simulink model "BCM2_4"  (R2021b)
settings: Solver=FixedStepDiscrete  StartTime=0.0  StopTime=1  FixedStep=0.001  RelTol=1e-3  EnableMultiTasking=on
InitFcn:
  | mbd_mpc_consistency_checks(bdroot(gcs));
model workspace (MAT data in the model file):
  CAN_rec : Simulink.Signal (value not decoded)
  CAN_transm_stat : Simulink.Signal (value not decoded)
  CAN_trm : Simulink.Signal (value not decoded)
  DITHER_CFB0 : Simulink.Parameter (value not decoded)
  DITHER_CFB1 : Simulink.Parameter (value not decoded)
  DITHER_CFB2 : Simulink.Parameter (value not decoded)
  DITHER_EN0 : Simulink.Parameter (value not decoded)
  DITHER_EN1 : Simulink.Parameter (value not decoded)
  DITHER_EN2 : Simulink.Parameter (value not decoded)
  DITHER_SIZE0 : Simulink.Parameter (value not decoded)
  DITHER_SIZE1 : Simulink.Parameter (value not decoded)
  DITHER_SIZE2 : Simulink.Parameter (value not decoded)
  DITHER_STEP0 : Simulink.Parameter (value not decoded)
  DITHER_STEP1 : Simulink.Parameter (value not decoded)
  DITHER_STEP2 : Simulink.Parameter (value not decoded)
  DITHER_SYNC0 : Simulink.Parameter (value not decoded)
  DITHER_SYNC1 : Simulink.Parameter (value not decoded)
  DITHER_SYNC2 : Simulink.Parameter (value not decoded)
  ECUMbut : Simulink.Signal (value not decoded)
  FAULTN : Simulink.Signal (value not decoded)
  FM0 : Simulink.Parameter (value not decoded)
  FM1 : Simulink.Parameter (value not decoded)
  FM2 : Simulink.Parameter (value not decoded)
  FME : Simulink.Parameter (value not decoded)
  Fsys_M : Simulink.Parameter (value not decoded)
  Fsys_N : Simulink.Parameter (value not decoded)
  Fsys_WDEN : Simulink.Parameter (value not decoded)
  Fsys_div : Simulink.Parameter (value not decoded)
  HL0 : Simulink.Parameter (value not decoded)
  HL1 : Simulink.Parameter (value not decoded)
  HL2 : Simulink.Parameter (value not decoded)
  IDIAG0 : Simulink.Parameter (value not decoded)
  IDIAG1 : Simulink.Parameter (value not decoded)
  IDIAG2 : Simulink.Parameter (value not decoded)
  Ivalve : Simulink.Signal (value not decoded)
  KI_index0 : Simulink.Parameter (value not decoded)
  KI_index1 : Simulink.Parameter (value not decoded)
  KI_index2 : Simulink.Parameter (value not decoded)
  PWM_Period0 : Simulink.Parameter (value not decoded)
  PWM_Period1 : Simulink.Parameter (value not decoded)
  PWM_Period2 : Simulink.Parameter (value not decoded)
  RESN : Simulink.Signal (value not decoded)
  SR0 : Simulink.Parameter (value not decoded)
  SR1 : Simulink.Parameter (value not decoded)
  SR2 : Simulink.Parameter (value not decoded)
  Vparam : Simulink.Signal (value not decoded)
  block_tle : Simulink.Signal (value not decoded)
  disp : Simulink.Signal (value not decoded)
  ee_adr : Simulink.Signal (value not decoded)
  ee_en_rd : Simulink.Signal (value not decoded)
  ee_en_wr : Simulink.Signal (value not decoded)
  ee_idle : Simulink.Signal (value not decoded)
  ee_read : Simulink.Signal (value not decoded)
  ee_recv : Simulink.Signal (value not decoded)
  ee_send : Simulink.Signal (value not decoded)
  in_stats : Simulink.Signal (value not decoded)
  inputs : Simulink.Signal (value not decoded)
  light : Simulink.Signal (value not decoded)
  out_drv : Simulink.Signal (value not decoded)
  out_drv_test : Simulink.Signal (value not decoded)
  out_test_en : Simulink.Signal (value not decoded)
  recv_spi2 : Simulink.Signal (value not decoded)
  ret : Simulink.Signal (value not decoded)
  spi_rcv_tle82453 : Simulink.Signal (value not decoded)
  tle82453_Ivlv : Simulink.Signal (value not decoded)
  tle82453_err : Simulink.Signal (value not decoded)
  tle82453_reset : Simulink.Signal (value not decoded)
  wtdg_CAN : Simulink.Signal (value not decoded)
symbols that are objects in the model workspace (value not decoded): CAN_rec, CAN_transm_stat, ECUMbut, inputs, Ivalve, out_drv_test, recv_spi2, ret, SR0, tle82453_Ivlv
undefined symbols (not defined in the file or in its folder): color, LQFP
libraries: simulink x68, mbd_mpc574x_ec_toolbox x50, canmsglib x42, hdlsllib x9, commutil2 x7, etargetslib x4
(part 2 of 6)

== system BCM2_4/Степы ретардера ==
  Data Store Write : DataStoreWrite  Commented=on  DataStoreName=ret  DataStoreElements=ret.step  IndexOptions=Index vector (dialog)  Indices=1  OutputSizes=1
  From2 : From  Commented=on  GotoTag=ret_stepM  TagVisibility=global
  From3 : From  Commented=on  GotoTag=ret_stepP  TagVisibility=global
  OR : Logic  Operator=OR  AllPortsSameDT=off  OutDataTypeStr=boolean
  eeprom степы ретардера : Stateflow chart  TreatAsAtomicUnit=on
      settings: PortSchema="{\"entries\":[{\"content\":{\"sides\":[{\"content\":{\"connectorIds\":[\"In1\",\"In3\",\"In2\"]},\"type\":\"ConnectorPlacement.EquallySpacedRectSide\",\"uuid\":\"1ebf9d07-d9d5-4765-a14b-d01132fae39d\"},{\"content\":{\"connectorIds\":[],\"side\":\"RIGHT\"},\"type\":\"ConnectorPlacement.EquallySpacedRectSide\",\"uuid\":\"961b2fe5-8f90-4192-8201-219491ef069e\"},{\"content\":{\"connectorIds\":[],\"side\":\"TOP\"},\"type\":\"ConnectorPlacement.EquallySpacedRectSide\",\"uuid\":\"9050879b-edec-4af7-9289-aadedb2c5dee\"}]},\"type\":\"ConnectorPlacement.EquallySpacedConnector\",\"uuid\":\"75c99b9c-2e9d-4193-9189-f6fceb65a5f8\"}],\"packageUris\":[\"http://schema.mathworks.com/mf0/Connector/R2020b\"],\"version\":\"1.0\"}"
  Степы ретардера : Stateflow chart  Commented=on  TreatAsAtomicUnit=on
  страницы механика+ : Subsystem  TreatAsAtomicUnit=on
  страницы механика- : Subsystem  TreatAsAtomicUnit=on
  wires:
  From2/1 -> Степы ретардера/1(stepM)
  Степы ретардера/1(Step_ret) -> Data Store Write/1
  From3/1 -> Степы ретардера/2(stepP)
  [ret_stepM] -> OR/1, страницы механика-/Trigger
  OR/1 -> eeprom степы ретардера/1(write_ee)
  [ret_stepP] -> страницы механика+/Trigger, OR/2
  страницы механика+/1(Out_max_ret) -> eeprom степы ретардера/3(step_max)
  страницы механика+/2(Out_max_brk) -> eeprom степы ретардера/2(step_brk_max)

== system BCM2_4/Топливные баки ==
  Pump1 : Inport
  Pump2 : Inport  Port=2
  rashod : Inport  Port=3
  Compare To Constant : simulink/Logic and Bit Operations/Compare To Constant  relop=>  const=0  OutDataTypeStr=boolean
  Data Store Memory : DataStoreMemory  DataStoreName=tank1  ReadBeforeWriteMsg=warning  WriteAfterWriteMsg=warning  WriteAfterReadMsg=warning  InitialValue=ft1  ShowAdditionalParam=off
  Data Store Memory1 : DataStoreMemory  DataStoreName=tank2  ReadBeforeWriteMsg=warning  WriteAfterWriteMsg=warning  WriteAfterReadMsg=warning  InitialValue=ft2  ShowAdditionalParam=off
  Data Store Memory2 : DataStoreMemory  DataStoreName=tank3  ReadBeforeWriteMsg=warning  WriteAfterWriteMsg=warning  WriteAfterReadMsg=warning  InitialValue=ft3  ShowAdditionalParam=off
  Data Store Read : DataStoreRead  DataStoreName=tank3  IndexOptions=Index vector (dialog)  Indices=1  OutputSizes=1
  Data Store Read4 : DataStoreRead  DataStoreName=tank1  IndexOptions=Index vector (dialog)  Indices=1  OutputSizes=1
  Data Store Read5 : DataStoreRead  DataStoreName=tank2  IndexOptions=Index vector (dialog)  Indices=1  OutputSizes=1
  Data Store Read6 : DataStoreRead  DataStoreName=tank3  IndexOptions=Index vector (dialog)  Indices=1  OutputSizes=1
  Enabled Subsystem : Subsystem  TreatAsAtomicUnit=on
  Enabled Subsystem1 : Subsystem  TreatAsAtomicUnit=on
  Subsystem : Subsystem
  Tank1 : Outport
  Tank2 : Outport  Port=2
  Tank3 : Outport  Port=3
  wires:
  Pump1/1 -> Enabled Subsystem/Enable
  Pump2/1 -> Enabled Subsystem1/Enable
  Data Store Read4/1 -> Tank1/1
  Data Store Read5/1 -> Tank2/1
  Data Store Read6/1 -> Tank3/1
  rashod/1 -> Subsystem/1(In1)
  Data Store Read/1 -> Compare To Constant/1
  Compare To Constant/1 -> Subsystem/Enable

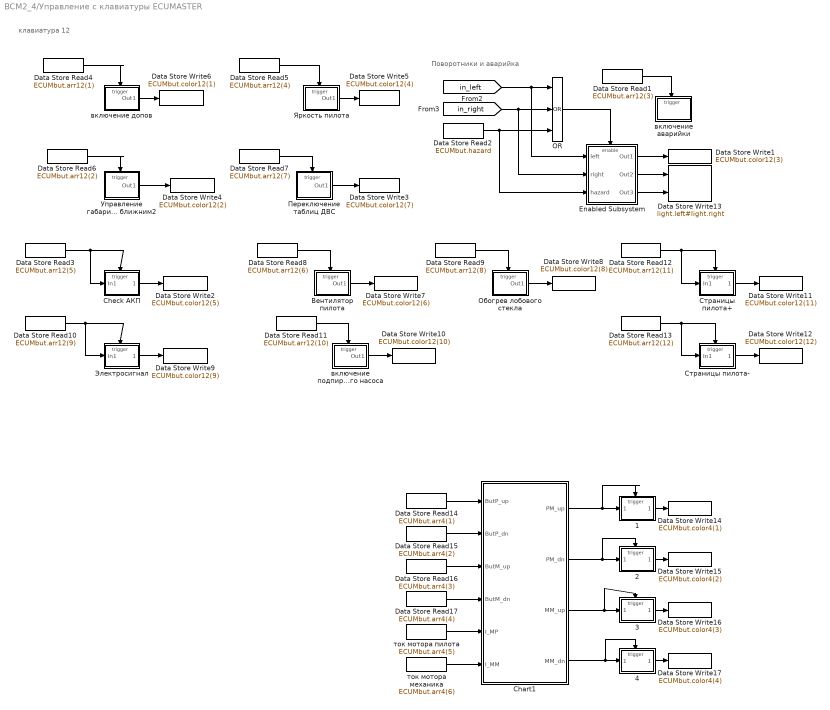
== system BCM2_4/Управление с клавиатуры ECUMASTER ==
  note: клавиатура 12
  note: Поворотники и аварийка
  1 : Subsystem
  2 : Subsystem
  3 : Subsystem
  4 : Subsystem
  Chart1 : Stateflow chart  TreatAsAtomicUnit=on
  Check АКП : Subsystem
  Data Store Read1 : DataStoreRead  DataStoreName=ECUMbut  DataStoreElements=ECUMbut.arr12(3)  IndexOptions=Index vector (dialog)  Indices=1  OutputSizes=1
  Data Store Read10 : DataStoreRead  DataStoreName=ECUMbut  DataStoreElements=ECUMbut.arr12(9)  IndexOptions=Index vector (dialog)  Indices=1  OutputSizes=1
  Data Store Read11 : DataStoreRead  DataStoreName=ECUMbut  DataStoreElements=ECUMbut.arr12(10)  IndexOptions=Index vector (dialog)  Indices=1  OutputSizes=1
  Data Store Read12 : DataStoreRead  DataStoreName=ECUMbut  DataStoreElements=ECUMbut.arr12(11)  IndexOptions=Index vector (dialog)  Indices=1  OutputSizes=1
  Data Store Read13 : DataStoreRead  DataStoreName=ECUMbut  DataStoreElements=ECUMbut.arr12(12)  IndexOptions=Index vector (dialog)  Indices=1  OutputSizes=1
  Data Store Read14 : DataStoreRead  DataStoreName=ECUMbut  DataStoreElements=ECUMbut.arr4(1)  IndexOptions=Index vector (dialog)  Indices=1  OutputSizes=1
  Data Store Read15 : DataStoreRead  DataStoreName=ECUMbut  DataStoreElements=ECUMbut.arr4(2)  IndexOptions=Index vector (dialog)  Indices=1  OutputSizes=1
  Data Store Read16 : DataStoreRead  DataStoreName=ECUMbut  DataStoreElements=ECUMbut.arr4(3)  IndexOptions=Index vector (dialog)  Indices=1  OutputSizes=1
  Data Store Read17 : DataStoreRead  DataStoreName=ECUMbut  DataStoreElements=ECUMbut.arr4(4)  IndexOptions=Index vector (dialog)  Indices=1  OutputSizes=1
  Data Store Read2 : DataStoreRead  DataStoreName=ECUMbut  DataStoreElements=ECUMbut.hazard  IndexOptions=Index vector (dialog)  Indices=1  OutputSizes=1
  Data Store Read3 : DataStoreRead  DataStoreName=ECUMbut  DataStoreElements=ECUMbut.arr12(5)  IndexOptions=Index vector (dialog)  Indices=1  OutputSizes=1
  Data Store Read4 : DataStoreRead  DataStoreName=ECUMbut  DataStoreElements=ECUMbut.arr12(1)  IndexOptions=Index vector (dialog)  Indices=1  OutputSizes=1
  Data Store Read5 : DataStoreRead  DataStoreName=ECUMbut  DataStoreElements=ECUMbut.arr12(4)  IndexOptions=Index vector (dialog)  Indices=1  OutputSizes=1
  Data Store Read6 : DataStoreRead  DataStoreName=ECUMbut  DataStoreElements=ECUMbut.arr12(2)  IndexOptions=Index vector (dialog)  Indices=1  OutputSizes=1
  Data Store Read7 : DataStoreRead  DataStoreName=ECUMbut  DataStoreElements=ECUMbut.arr12(7)  IndexOptions=Index vector (dialog)  Indices=1  OutputSizes=1
  Data Store Read8 : DataStoreRead  DataStoreName=ECUMbut  DataStoreElements=ECUMbut.arr12(6)  IndexOptions=Index vector (dialog)  Indices=1  OutputSizes=1
  Data Store Read9 : DataStoreRead  DataStoreName=ECUMbut  DataStoreElements=ECUMbut.arr12(8)  IndexOptions=Index vector (dialog)  Indices=1  OutputSizes=1
  Data Store Write1 : DataStoreWrite  DataStoreName=ECUMbut  DataStoreElements=ECUMbut.color12(3)  IndexOptions=Index vector (dialog)  Indices=1  OutputSizes=1
  Data Store Write10 : DataStoreWrite  DataStoreName=ECUMbut  DataStoreElements=ECUMbut.color12(10)  IndexOptions=Index vector (dialog)  Indices=1  OutputSizes=1
  Data Store Write11 : DataStoreWrite  DataStoreName=ECUMbut  DataStoreElements=ECUMbut.color12(11)  IndexOptions=Index vector (dialog)  Indices=1  OutputSizes=1
  Data Store Write12 : DataStoreWrite  DataStoreName=ECUMbut  DataStoreElements=ECUMbut.color12(12)  IndexOptions=Index vector (dialog)  Indices=1  OutputSizes=1
  Data Store Write13 : DataStoreWrite  DataStoreName=light  DataStoreElements=light.left#light.right  IndexOptions=Index vector (dialog)  Indices=1  OutputSizes=1
  Data Store Write14 : DataStoreWrite  DataStoreName=ECUMbut  DataStoreElements=ECUMbut.color4(1)  IndexOptions=Index vector (dialog)  Indices=1  OutputSizes=1
  Data Store Write15 : DataStoreWrite  DataStoreName=ECUMbut  DataStoreElements=ECUMbut.color4(2)  IndexOptions=Index vector (dialog)  Indices=1  OutputSizes=1
  Data Store Write16 : DataStoreWrite  DataStoreName=ECUMbut  DataStoreElements=ECUMbut.color4(3)  IndexOptions=Index vector (dialog)  Indices=1  OutputSizes=1
  Data Store Write17 : DataStoreWrite  DataStoreName=ECUMbut  DataStoreElements=ECUMbut.color4(4)  IndexOptions=Index vector (dialog)  Indices=1  OutputSizes=1
  Data Store Write2 : DataStoreWrite  DataStoreName=ECUMbut  DataStoreElements=ECUMbut.color12(5)  IndexOptions=Index vector (dialog)  Indices=1  OutputSizes=1
  Data Store Write3 : DataStoreWrite  DataStoreName=ECUMbut  DataStoreElements=ECUMbut.color12(7)  IndexOptions=Index vector (dialog)  Indices=1  OutputSizes=1
  Data Store Write4 : DataStoreWrite  DataStoreName=ECUMbut  DataStoreElements=ECUMbut.color12(2)  IndexOptions=Index vector (dialog)  Indices=1  OutputSizes=1
  Data Store Write5 : DataStoreWrite  DataStoreName=ECUMbut  DataStoreElements=ECUMbut.color12(4)  IndexOptions=Index vector (dialog)  Indices=1  OutputSizes=1
  Data Store Write6 : DataStoreWrite  DataStoreName=ECUMbut  DataStoreElements=ECUMbut.color12(1)  IndexOptions=Index vector (dialog)  Indices=1  OutputSizes=1
  Data Store Write7 : DataStoreWrite  DataStoreName=ECUMbut  DataStoreElements=ECUMbut.color12(6)  IndexOptions=Index vector (dialog)  Indices=1  OutputSizes=1
  Data Store Write8 : DataStoreWrite  DataStoreName=ECUMbut  DataStoreElements=ECUMbut.color12(8)  IndexOptions=Index vector (dialog)  Indices=1  OutputSizes=1
  Data Store Write9 : DataStoreWrite  DataStoreName=ECUMbut  DataStoreElements=ECUMbut.color12(9)  IndexOptions=Index vector (dialog)  Indices=1  OutputSizes=1
  Enabled Subsystem : Subsystem  TreatAsAtomicUnit=on
  OR : Logic  Operator=OR  Inputs=3  AllPortsSameDT=off  OutDataTypeStr=boolean
  Вентилятор пилота : Subsystem
  Обогрев лобового стекла : Subsystem
  Переключение таблиц ДВС : Subsystem  TreatAsAtomicUnit=on
  Страницы пилота+ : Subsystem
  Страницы пилота- : Subsystem
  Управление габаритами и ближним2 : Subsystem  TreatAsAtomicUnit=on
  Электросигнал : Subsystem
  Яркость пилота : Subsystem
  включение аварийки : Subsystem
  включение допов : Subsystem
  включение подпирающего топливного насоса : Subsystem
  ток мотора механика : DataStoreRead  DataStoreName=ECUMbut  DataStoreElements=ECUMbut.arr4(6)  IndexOptions=Index vector (dialog)  Indices=1  OutputSizes=1
  ток мотора пилота : DataStoreRead  DataStoreName=ECUMbut  DataStoreElements=ECUMbut.arr4(5)  IndexOptions=Index vector (dialog)  Indices=1  OutputSizes=1
  wires:
  Data Store Read4/1 -> включение допов/Trigger
  Яркость пилота/1(Out1) -> Data Store Write5/1
  Data Store Read7/1 -> Переключение таблиц ДВС/Trigger
  Data Store Read5/1 -> Яркость пилота/Trigger
  Управление габаритами и ближним2/1(Out1) -> Data Store Write4/1
  включение допов/1(Out1) -> Data Store Write6/1
  Переключение таблиц ДВС/1(Out1) -> Data Store Write3/1
  Data Store Read6/1 -> Управление габаритами и ближним2/Trigger
  Data Store Read1/1 -> включение аварийки/Trigger
  [in_left] -> Enabled Subsystem/1(left), OR/1
  [in_right] -> Enabled Subsystem/2(right), OR/2
  Data Store Read2/1 -> Enabled Subsystem/3(hazard), OR/3
  OR/1 -> Enabled Subsystem/Enable
  Enabled Subsystem/1(Out1) -> Data Store Write1/1
  Check АКП/1(Out1) -> Data Store Write2/1
  Data Store Read3/1 -> Check АКП/1(In1), Check АКП/Trigger
  Вентилятор пилота/1(Out1) -> Data Store Write7/1
  Data Store Read8/1 -> Вентилятор пилота/Trigger
  Обогрев лобового стекла/1(Out1) -> Data Store Write8/1
  Data Store Read9/1 -> Обогрев лобового стекла/Trigger
  Data Store Read10/1 -> Электросигнал/1(In1), Электросигнал/Trigger
  Электросигнал/1(Out1) -> Data Store Write9/1
  включение подпирающего топливного насоса/1(Out1) -> Data Store Write10/1
  Data Store Read11/1 -> включение подпирающего топливного насоса/Trigger
  Страницы пилота+/1(Out1) -> Data Store Write11/1
  Data Store Read12/1 -> Страницы пилота+/Trigger, Страницы пилота+/1(In1)
  Data Store Read13/1 -> Страницы пилота-/1(In1), Страницы пилота-/Trigger
  Страницы пилота-/1(Out1) -> Data Store Write12/1
  Enabled Subsystem/2(Out2) -> Data Store Write13/1
  Enabled Subsystem/3(Out3) -> Data Store Write13/2
  1/1(Out1) -> Data Store Write14/1
  ток мотора пилота/1 -> Chart1/5(I_MP)
  ток мотора механика/1 -> Chart1/6(I_MM)
  Chart1/1(PM_up) -> 1/1(PM_up), 1/Trigger
  2/1(Out1) -> Data Store Write15/1
  3/1(Out1) -> Data Store Write16/1
  4/1(Out1) -> Data Store Write17/1
  Chart1/2(PM_dn) -> 2/Trigger, 2/1(PM_up)
  Chart1/3(MM_up) -> 3/1(PM_up), 3/Trigger
  Chart1/4(MM_dn) -> 4/1(PM_up), 4/Trigger
  Data Store Read14/1 -> Chart1/1(ButP_up)
  Data Store Read15/1 -> Chart1/2(ButP_dn)
  Data Store Read16/1 -> Chart1/3(ButM_up)
  Data Store Read17/1 -> Chart1/4(ButM_dn)

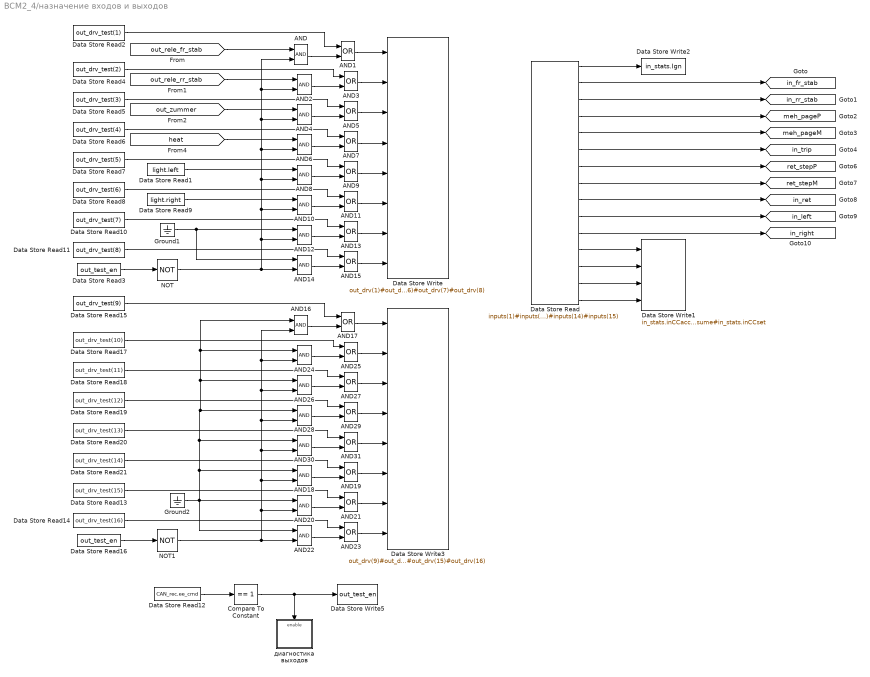
== system BCM2_4/назначение входов и выходов ==
  AND{,2,4,6,8,10,12,14,16,18,20,22,24,26,28,30} (16 alike) : Logic  AllPortsSameDT=off  OutDataTypeStr=boolean
  AND{1,3,5,7,9,11,13,15,17,19,21,23,25,27,29,31} (16 alike) : Logic  Operator=OR  AllPortsSameDT=off  OutDataTypeStr=boolean
  Compare To Constant : simulink/Logic and Bit Operations/Compare To Constant  relop===  const=1  OutDataTypeStr=boolean
  Data Store Read : DataStoreRead  DataStoreName=inputs  DataStoreElements=inputs(1)#inputs(2)#inputs(3)#inputs(4)#inputs(5)#inputs(6)#inputs(7)#inputs(8)#inputs(9)#inputs(10)#inputs(11)#inputs(12)#inputs(13)#inputs(14)#inputs(15)  IndexOptions=Index vector (dialog)  Indices=1  OutputSizes=1
  Data Store Read1 : DataStoreRead  DataStoreName=light  DataStoreElements=light.left  IndexOptions=Index vector (dialog)  Indices=1  OutputSizes=1
  Data Store Read10 : DataStoreRead  DataStoreName=out_drv_test  DataStoreElements=out_drv_test(7)  IndexOptions=Index vector (dialog)  Indices=1  OutputSizes=1
  Data Store Read11 : DataStoreRead  DataStoreName=out_drv_test  DataStoreElements=out_drv_test(8)  IndexOptions=Index vector (dialog)  Indices=1  OutputSizes=1
  Data Store Read12 : DataStoreRead  DataStoreName=CAN_rec  SampleTime=0.1  DataStoreElements=CAN_rec.ee_cmd  IndexOptions=Index vector (dialog)  Indices=1  OutputSizes=1
  Data Store Read13 : DataStoreRead  DataStoreName=out_drv_test  DataStoreElements=out_drv_test(15)  IndexOptions=Index vector (dialog)  Indices=1  OutputSizes=1
  Data Store Read14 : DataStoreRead  DataStoreName=out_drv_test  DataStoreElements=out_drv_test(16)  IndexOptions=Index vector (dialog)  Indices=1  OutputSizes=1
  Data Store Read15 : DataStoreRead  DataStoreName=out_drv_test  DataStoreElements=out_drv_test(9)  IndexOptions=Index vector (dialog)  Indices=1  OutputSizes=1
  Data Store Read16 : DataStoreRead  DataStoreName=out_test_en  IndexOptions=Index vector (dialog)  Indices=1  OutputSizes=1
  Data Store Read17 : DataStoreRead  DataStoreName=out_drv_test  DataStoreElements=out_drv_test(10)  IndexOptions=Index vector (dialog)  Indices=1  OutputSizes=1
  Data Store Read18 : DataStoreRead  DataStoreName=out_drv_test  DataStoreElements=out_drv_test(11)  IndexOptions=Index vector (dialog)  Indices=1  OutputSizes=1
  Data Store Read19 : DataStoreRead  DataStoreName=out_drv_test  DataStoreElements=out_drv_test(12)  IndexOptions=Index vector (dialog)  Indices=1  OutputSizes=1
  Data Store Read2 : DataStoreRead  DataStoreName=out_drv_test  DataStoreElements=out_drv_test(1)  IndexOptions=Index vector (dialog)  Indices=1  OutputSizes=1
  Data Store Read20 : DataStoreRead  DataStoreName=out_drv_test  DataStoreElements=out_drv_test(13)  IndexOptions=Index vector (dialog)  Indices=1  OutputSizes=1
  Data Store Read21 : DataStoreRead  DataStoreName=out_drv_test  DataStoreElements=out_drv_test(14)  IndexOptions=Index vector (dialog)  Indices=1  OutputSizes=1
  Data Store Read3 : DataStoreRead  DataStoreName=out_test_en  IndexOptions=Index vector (dialog)  Indices=1  OutputSizes=1
  Data Store Read4 : DataStoreRead  DataStoreName=out_drv_test  DataStoreElements=out_drv_test(2)  IndexOptions=Index vector (dialog)  Indices=1  OutputSizes=1
  Data Store Read5 : DataStoreRead  DataStoreName=out_drv_test  DataStoreElements=out_drv_test(3)  IndexOptions=Index vector (dialog)  Indices=1  OutputSizes=1
  Data Store Read6 : DataStoreRead  DataStoreName=out_drv_test  DataStoreElements=out_drv_test(4)  IndexOptions=Index vector (dialog)  Indices=1  OutputSizes=1
  Data Store Read7 : DataStoreRead  DataStoreName=out_drv_test  DataStoreElements=out_drv_test(5)  IndexOptions=Index vector (dialog)  Indices=1  OutputSizes=1
  Data Store Read8 : DataStoreRead  DataStoreName=out_drv_test  DataStoreElements=out_drv_test(6)  IndexOptions=Index vector (dialog)  Indices=1  OutputSizes=1
  Data Store Read9 : DataStoreRead  DataStoreName=light  DataStoreElements=light.right  IndexOptions=Index vector (dialog)  Indices=1  OutputSizes=1
  Data Store Write : DataStoreWrite  DataStoreName=out_drv  DataStoreElements=out_drv(1)#out_drv(2)#out_drv(3)#out_drv(4)#out_drv(5)#out_drv(6)#out_drv(7)#out_drv(8)  IndexOptions=Index vector (dialog)  Indices=1  OutputSizes=1
  Data Store Write1 : DataStoreWrite  DataStoreName=in_stats  DataStoreElements=in_stats.inCCacc#in_stats.inCCcoast#in_stats.inCCresume#in_stats.inCCset  IndexOptions=Index vector (dialog)  Indices=1  OutputSizes=1
  Data Store Write2 : DataStoreWrite  DataStoreName=in_stats  DataStoreElements=in_stats.Ign  IndexOptions=Index vector (dialog)  Indices=1  OutputSizes=1
  Data Store Write3 : DataStoreWrite  DataStoreName=out_drv  SampleTime=0.01  DataStoreElements=out_drv(9)#out_drv(10)#out_drv(11)#out_drv(12)#out_drv(13)#out_drv(14)#out_drv(15)#out_drv(16)  IndexOptions=Index vector (dialog)  Indices=1  OutputSizes=1
  Data Store Write5 : DataStoreWrite  DataStoreName=out_test_en  IndexOptions=Index vector (dialog)  Indices=1  OutputSizes=1
  Ground1 : Ground
  Ground2 : Ground
  NOT : Logic  Operator=NOT  IconShape=distinctive  AllPortsSameDT=off  OutDataTypeStr=boolean
  NOT1 : Logic  Operator=NOT  IconShape=distinctive  AllPortsSameDT=off  OutDataTypeStr=boolean
  диагностика выходов : Subsystem
  tag scope: in_fr_stab=global, in_left=global, in_ret=global, in_right=global, in_rr_stab=global, in_trip=global, meh_pageM=global, meh_pageP=global, ret_stepM=global, ret_stepP=global
  wires:
  Data Store Read/5 -> [meh_pageM]
  Data Store Read/6 -> [in_trip]
  Data Store Read/7 -> [ret_stepP]
  Data Store Read/8 -> [ret_stepM]
  Data Store Read/9 -> [in_ret]
  Data Store Read/10 -> [in_left]
  Data Store Read/11 -> [in_right]
  [out_rele_fr_stab] -> AND/1
  [out_rele_rr_stab] -> AND2/1
  [out_zummer] -> AND4/1
  Ground1/1 -> AND12/1, AND14/1
  [heat] -> AND6/1
  Data Store Read1/1 -> AND8/1
  Data Store Read9/1 -> AND10/1
  Data Store Read/12 -> Data Store Write1/1
  Data Store Read/13 -> Data Store Write1/2
  Data Store Read/14 -> Data Store Write1/3
  Data Store Read/15 -> Data Store Write1/4
  Data Store Read/1 -> Data Store Write2/1
  Data Store Read/2 -> [in_fr_stab]
  Data Store Read/3 -> [in_rr_stab]
  Data Store Read/4 -> [meh_pageP]
  AND1/1 -> Data Store Write/1
  AND/1 -> AND1/2
  AND2/1 -> AND3/2
  AND3/1 -> Data Store Write/2
  AND4/1 -> AND5/2
  AND5/1 -> Data Store Write/3
  AND6/1 -> AND7/2
  AND7/1 -> Data Store Write/4
  AND8/1 -> AND9/2
  AND9/1 -> Data Store Write/5
  AND10/1 -> AND11/2
  AND11/1 -> Data Store Write/6
  AND12/1 -> AND13/2
  AND13/1 -> Data Store Write/7
  AND14/1 -> AND15/2
  AND15/1 -> Data Store Write/8
  Data Store Read3/1 -> NOT/1
  Data Store Read2/1 -> AND1/1
  Data Store Read4/1 -> AND3/1
  Data Store Read5/1 -> AND5/1
  Data Store Read6/1 -> AND7/1
  Data Store Read7/1 -> AND9/1
  Data Store Read8/1 -> AND11/1
  Data Store Read10/1 -> AND13/1
  Data Store Read11/1 -> AND15/1
  Data Store Read14/1 -> AND23/1
  Data Store Read13/1 -> AND21/1
  Data Store Read21/1 -> AND19/1
  Data Store Read20/1 -> AND31/1
  Data Store Read19/1 -> AND29/1
  Data Store Read18/1 -> AND27/1
  Data Store Read17/1 -> AND25/1
  Data Store Read15/1 -> AND17/1
  Data Store Read16/1 -> NOT1/1
  AND23/1 -> Data Store Write3/8
  AND22/1 -> AND23/2
  AND21/1 -> Data Store Write3/7
  AND20/1 -> AND21/2
  AND19/1 -> Data Store Write3/6
  AND18/1 -> AND19/2
  AND31/1 -> Data Store Write3/5
  AND30/1 -> AND31/2
  AND29/1 -> Data Store Write3/4
  AND28/1 -> AND29/2
  AND27/1 -> Data Store Write3/3
  AND26/1 -> AND27/2
  AND25/1 -> Data Store Write3/2
  AND24/1 -> AND25/2
  AND16/1 -> AND17/2
  AND17/1 -> Data Store Write3/1
  Ground2/1 -> AND22/1, AND16/1, AND24/1, AND26/1, AND28/1, AND30/1, AND18/1, AND20/1
  NOT/1 -> AND14/2, AND12/2, AND10/2, AND8/2, AND6/2, AND4/2, AND2/2, AND/2
  NOT1/1 -> AND16/2, AND24/2, AND26/2, AND28/2, AND30/2, AND18/2, AND20/2, AND22/2
  Compare To Constant/1 -> Data Store Write5/1, диагностика выходов/Enable
  Data Store Read12/1 -> Compare To Constant/1

== system BCM2_4/управление лепестками ==
  Data Store Write : DataStoreWrite  DataStoreName=ret  DataStoreElements=ret.ret_en  IndexOptions=Index vector (dialog)  Indices=1  OutputSizes=1
  Remote stab : Stateflow chart  TreatAsAtomicUnit=on
  tag scope: out_rele_fr_stab=global, out_rele_rr_stab=global, out_zummer=global
  wires:
  [in_fr_stab] -> Remote stab/1(sw_fr_stab)
  Remote stab/3(zummer) -> [out_zummer]
  Remote stab/2(rele_rr_stab) -> [out_rele_rr_stab]
  Remote stab/1(rele_fr_stab) -> [out_rele_fr_stab]
  [in_rr_stab] -> Remote stab/2(sw_rr_stab)
  Remote stab/4(rele_ret) -> Data Store Write/1
  [in_ret] -> Remote stab/3(sw_ret)

== system BCM2_4/управление страницами и яркостью мониторов ==
  Constant : Constant  OutDataTypeStr=boolean
  Data Store Read1 : DataStoreRead  DataStoreName=ECUMbut  DataStoreElements=ECUMbut.bright_pilot  IndexOptions=Index vector (dialog)  Indices=1  OutputSizes=1
  Data Store Read2 : DataStoreRead  DataStoreName=CAN_trm  DataStoreElements=CAN_trm.wPilotPageP#CAN_trm.wPilotPageM  IndexOptions=Index vector (dialog)  Indices=1  OutputSizes=1
  Data Store Read4 : DataStoreRead  DataStoreName=ECUMbut  DataStoreElements=ECUMbut.PageP#ECUMbut.PageM  IndexOptions=Index vector (dialog)  Indices=1  OutputSizes=1
  Display : Display
  Display1 : Display
  OR : Logic  Operator=OR  Inputs=4  AllPortsSameDT=off  OutDataTypeStr=boolean
  OR1 : Logic  Operator=OR  AllPortsSameDT=off  OutDataTypeStr=boolean
  OR2 : Logic  Operator=OR  AllPortsSameDT=off  OutDataTypeStr=boolean
  Remote bright : Stateflow chart  TreatAsAtomicUnit=on
      settings: PortSchema="{\"entries\":[{\"content\":{\"sides\":[{\"content\":{\"connectorIds\":[\"In2\",\"In1\"]},\"type\":\"ConnectorPlacement.EquallySpacedRectSide\",\"uuid\":\"b649a9c8-237f-4f0e-8c49-622a9c826017\"},{\"content\":{\"connectorIds\":[\"Out1\",\"Out2\"],\"side\":\"RIGHT\"},\"type\":\"ConnectorPlacement.EquallySpacedRectSide\",\"uuid\":\"0d804784-30f9-473e-82b5-002cce05e2f2\"},{\"content\":{\"connectorIds\":[],\"side\":\"TOP\"},\"type\":\"ConnectorPlacement.EquallySpacedRectSide\",\"uuid\":\"6d8957c1-8347-4a30-84c4-fd66e5fe6d42\"},{\"content\":{\"connectorIds\":[],\"side\":\"HIDDEN\"},\"type\":\"ConnectorPlacement.EquallySpacedRectSide\",\"uuid\":\"9712d6bb-fd29-4f07-870a-122e6c317742\"}]},\"type\":\"ConnectorPlacement.EquallySpacedConnector\",\"uuid\":\"dcd1749c-602d-455d-8651-1ffb4d1b2b2f\"}],\"packageUris\":[\"http://schema.mathworks.com/mf0/Connector/R2020b\"],\"version\":\"1.0\"}"
  eeprom страницы : Stateflow chart  TreatAsAtomicUnit=on
  страницы механика+ : Subsystem  TreatAsAtomicUnit=on
  страницы механика- : Subsystem  TreatAsAtomicUnit=on
  страницы пилота+ : Subsystem  TreatAsAtomicUnit=on
  страницы пилота- : Subsystem  TreatAsAtomicUnit=on
  wires:
  Constant/1 -> Remote bright/1(inM)
  Remote bright/1(outP) -> Display/1
  Remote bright/2(outM) -> Display1/1
  Data Store Read1/1 -> Remote bright/2(inP)
  [meh_pageP] -> страницы механика+/Trigger, OR/3
  [meh_pageM] -> страницы механика-/Trigger, OR/4
  OR2/1 -> страницы пилота-/Trigger, OR/2
  OR/1 -> eeprom страницы/1(write_ee)
  OR1/1 -> страницы пилота+/Trigger, OR/1
  Data Store Read4/1 -> OR1/2
  Data Store Read2/1 -> OR1/1
  Data Store Read4/2 -> OR2/1
  Data Store Read2/2 -> OR2/2

== system BCM2_4/CAN WATCHDOG/wtdg CCVS1_00 ==
  function : TriggerPort  TriggerType=function-call  VariantControl=(inherit)
  Constant : Constant  Value=0
  Data Store Write4 : DataStoreWrite  DataStoreName=Vparam  DataStoreElements=Vparam.Vspd  IndexOptions=Index vector (dialog)  Indices=1  OutputSizes=1
  wires:
  Constant/1 -> Data Store Write4/1

== system BCM2_4/CAN WATCHDOG/wtdg EBC1 ==
  function : TriggerPort  TriggerType=function-call  VariantControl=(inherit)
  Constant : Constant  Value=0  OutDataTypeStr=uint8
  Data Store Write : DataStoreWrite  DataStoreName=Vparam  DataStoreElements=Vparam.BrakePos  IndexOptions=Index vector (dialog)  Indices=1  OutputSizes=1
  wires:
  Constant/1 -> Data Store Write/1

== system BCM2_4/CAN WATCHDOG/wtdg EEC1_300 ==
  function : TriggerPort  TriggerType=function-call  VariantControl=(inherit)
  Constant : Constant  Value=0  OutDataTypeStr=uint8
  Data Store Write : DataStoreWrite  DataStoreName=Vparam  DataStoreElements=Vparam.PedalPos  IndexOptions=Index vector (dialog)  Indices=1  OutputSizes=1
  wires:
  Constant/1 -> Data Store Write/1

== system BCM2_4/CAN WATCHDOG/wtdg EEC1_400 ==
  function : TriggerPort  TriggerType=function-call  VariantControl=(inherit)
  Constant : Constant  Value=0  OutDataTypeStr=uint16
  Data Store Write : DataStoreWrite  DataStoreName=Vparam  DataStoreElements=Vparam.Espd  IndexOptions=Index vector (dialog)  Indices=1  OutputSizes=1
  wires:
  Constant/1 -> Data Store Write/1

== system BCM2_4/CAN WATCHDOG/wtdg ETC1 ==
  function : TriggerPort  TriggerType=function-call  VariantControl=(inherit)

== system BCM2_4/CAN WATCHDOG/wtdg FuelTank ==
  function : TriggerPort  TriggerType=function-call  VariantControl=(inherit)

== system BCM2_4/CAN WATCHDOG/wtdg RF ==
  function : TriggerPort  TriggerType=function-call  VariantControl=(inherit)
  Constant : Constant  Value=180
  Data Store Write : DataStoreWrite  DataStoreName=ret  DataStoreElements=ret.RetTemp  IndexOptions=Index vector (dialog)  Indices=1  OutputSizes=1
  wires:
  Constant/1 -> Data Store Write/1

== system BCM2_4/CAN WATCHDOG/wtdg VD ==
  function : TriggerPort  TriggerType=function-call  VariantControl=(inherit)

== system BCM2_4/CAN WATCHDOG/wtdg ee_wr ==
  function : TriggerPort  TriggerType=function-call  VariantControl=(inherit)
  Constant1 : Constant  Value=0  OutDataTypeStr=boolean
  Constant2 : Constant  Value=0  OutDataTypeStr=uint8
  Data Store Write2 : DataStoreWrite  DataStoreName=CAN_rec  DataStoreElements=CAN_rec.ee_rec_stat  IndexOptions=Index vector (dialog)  Indices=1  OutputSizes=1
  Data Store Write4 : DataStoreWrite  DataStoreName=CAN_rec  DataStoreElements=CAN_rec.ee_cmd  IndexOptions=Index vector (dialog)  Indices=1  OutputSizes=1
  wires:
  Constant1/1 -> Data Store Write2/1
  Constant2/1 -> Data Store Write4/1

== system BCM2_4/CAN WATCHDOG/wtdg id101 ==
  function : TriggerPort  TriggerType=function-call  VariantControl=(inherit)

== system BCM2_4/CAN WATCHDOG/wtdg id192 ==
  function : TriggerPort  TriggerType=function-call  VariantControl=(inherit)

== system BCM2_4/CAN WATCHDOG/wtdg id195 ==
  function : TriggerPort  TriggerType=function-call  VariantControl=(inherit)
  Constant : Constant  Value=[0 0 0 0 0 0 0 0 0 0 0 0 0 0 0 0]  OutDataTypeStr=boolean
  Data Store Write : DataStoreWrite  DataStoreName=ECUMbut  DataStoreElements=ECUMbut.arr12(:)  IndexOptions=Index vector (dialog)  Indices=1  OutputSizes=1
  wires:
  Constant/1 -> Data Store Write/1

== system BCM2_4/CAN WATCHDOG/wtdg max_page_meh ==
  function : TriggerPort  TriggerType=function-call  VariantControl=(inherit)

== system BCM2_4/CAN WATCHDOG/wtdg max_page_pilot ==
  function : TriggerPort  TriggerType=function-call  VariantControl=(inherit)

== system BCM2_4/CAN WATCHDOG/wtdg w18F0010B ==
  function : TriggerPort  TriggerType=function-call  VariantControl=(inherit)

== system BCM2_4/CAN WATCHDOG/wtdg w18FEAD0B ==
  function : TriggerPort  TriggerType=function-call  VariantControl=(inherit)

== system BCM2_4/CAN WATCHDOG/wtdg w18FEEA2F ==
  function : TriggerPort  TriggerType=function-call  VariantControl=(inherit)

== system BCM2_4/CAN0 Transmit buf 5-21/0CFED911 AUXIO buf = 11 ==
  Enable : EnablePort
  0CFED911 AUXIO buf = 11 : Subsystem  TreatAsAtomicUnit=on  SystemSampleTime=0.1

== system BCM2_4/CAN0 Transmit buf 5-21/0CFEF111 CCVS1 buf = 10 ==
  Enable : EnablePort
  0CFEF111 CCVS1 buf = 10 : Subsystem  TreatAsAtomicUnit=on  SystemSampleTime=0.1

== system BCM2_4/CAN0 Transmit buf 5-21/0x18FEF461 Чтение//Запись EEPROM buf = 6 ==
  Enable : EnablePort
  EBC1 0x18F0010B buf = 6 : Subsystem  TreatAsAtomicUnit=on  SystemSampleTime=0.001

== system BCM2_4/CAN0 Transmit buf 5-21/181112F2 Статусы buf = 5 ==
  Enable : EnablePort
  181112F2 статусы buf = 5 : Subsystem  TreatAsAtomicUnit=on  SystemSampleTime=0.1

== system BCM2_4/CAN0 Transmit buf 5-21/18F0010B buf = 7 ==
  Enable : EnablePort
  18F0010B buf = 7 : Subsystem  TreatAsAtomicUnit=on  SystemSampleTime=0.1

== system BCM2_4/CAN0 Transmit buf 5-21/18FEAD0B buf = 8 ==
  Enable : EnablePort
  18FEAD0B buf = 8 : Subsystem  TreatAsAtomicUnit=on  SystemSampleTime=0.1

== system BCM2_4/CAN0 Transmit buf 5-21/18FEEA2F buf = 9 ==
  Enable : EnablePort
  18FEEA2F buf = 9 : Subsystem  TreatAsAtomicUnit=on  SystemSampleTime=0.1

== system BCM2_4/CAN0 Transmit buf 5-21/Tx_Complete ==
  In1 : Inport
  function : TriggerPort  TriggerType=function-call  VariantControl=Variant
  If Action Subsystem1 : Subsystem  TreatAsAtomicUnit=on
  If Action Subsystem2 : Subsystem  TreatAsAtomicUnit=on
  If Action Subsystem3 : Subsystem  TreatAsAtomicUnit=on
  If Action Subsystem4 : Subsystem  TreatAsAtomicUnit=on
  If Action Subsystem5 : Subsystem  TreatAsAtomicUnit=on
  If Action Subsystem6 : Subsystem  TreatAsAtomicUnit=on
  If Action Subsystem7 : Subsystem  TreatAsAtomicUnit=on
  If Action Subsystem8 : Subsystem  TreatAsAtomicUnit=on
  Switch Case : SwitchCase  CaseConditions={5 6 7 8 9 10 11}
  wires:
  Switch Case/8 -> If Action Subsystem2/Action
  Switch Case/2 -> If Action Subsystem7/Action
  Switch Case/1 -> If Action Subsystem8/Action
  In1/1 -> Switch Case/1
  Switch Case/3 -> If Action Subsystem1/Action
  Switch Case/4 -> If Action Subsystem3/Action
  Switch Case/5 -> If Action Subsystem4/Action
  Switch Case/6 -> If Action Subsystem5/Action
  Switch Case/7 -> If Action Subsystem6/Action

== system BCM2_4/CAN1 Transmit buf 27-43/Tx_Complete ==
  In1 : Inport
  function : TriggerPort  TriggerType=function-call  VariantControl=Variant
  If Action Subsystem1 : Subsystem  TreatAsAtomicUnit=on
  If Action Subsystem2 : Subsystem  TreatAsAtomicUnit=on
  If Action Subsystem3 : Subsystem  TreatAsAtomicUnit=on
  If Action Subsystem4 : Subsystem  TreatAsAtomicUnit=on
  If Action Subsystem7 : Subsystem  TreatAsAtomicUnit=on
  If Action Subsystem8 : Subsystem  TreatAsAtomicUnit=on
  Switch Case : SwitchCase  CaseConditions={27 28 29 30 31}
  wires:
  In1/1 -> Switch Case/1
  Switch Case/1 -> If Action Subsystem8/Action
  Switch Case/2 -> If Action Subsystem7/Action
  Switch Case/6 -> If Action Subsystem2/Action
  Switch Case/3 -> If Action Subsystem1/Action
  Switch Case/4 -> If Action Subsystem3/Action
  Switch Case/5 -> If Action Subsystem4/Action

== system BCM2_4/CAN1 Transmit buf 27-43/Активация клавиатуры buf = 27 ==
  Enable : EnablePort
  Активация клавиатуры buf = 27 : Subsystem  TreatAsAtomicUnit=on  SystemSampleTime=1

== system BCM2_4/CAN1 Transmit buf 27-43/Цвет клавиатуры 12 buf = 28 ==
  Enable : EnablePort
  Цвет клавиатуры buf = 28 : Subsystem  TreatAsAtomicUnit=on  SystemSampleTime=0.1

== system BCM2_4/CAN1 Transmit buf 27-43/Цвет клавиатуры 4 buf = 30 ==
  Enable : EnablePort
  Цвет клавиатуры buf = 30 : Subsystem  TreatAsAtomicUnit=on  SystemSampleTime=0.1

== system BCM2_4/CAN1 Transmit buf 27-43/подсветка клавиатуры buf = 29 ==
  Enable : EnablePort
  подсветка клавиатуры buf = 29 : Subsystem  TreatAsAtomicUnit=on  SystemSampleTime=0.5

== system BCM2_4/CAN1 Transmit buf 27-43/подсветка клавиатуры buf = 31 ==
  Enable : EnablePort
  подсветка клавиатуры buf = 31 : Subsystem  TreatAsAtomicUnit=on  SystemSampleTime=0.5

== system BCM2_4/CAN2 Transmit buf 49-59/EBC1 0x18F0010D Педаль тормоза buf = 9 ==
  Enable : EnablePort
  EBC1 0x18F0010D buf = 9 : Subsystem  TreatAsAtomicUnit=on  SystemSampleTime=0.1

== system BCM2_4/CAN2 Transmit buf 49-59/Tx_Complete ==
  In1 : Inport
  function : TriggerPort  TriggerType=function-call  VariantControl=Variant
  If Action Subsystem2 : Subsystem  TreatAsAtomicUnit=on
  If Action Subsystem7 : Subsystem  TreatAsAtomicUnit=on
  If Action Subsystem8 : Subsystem  TreatAsAtomicUnit=on
  Switch Case : SwitchCase  CaseConditions={9 21}
  wires:
  Switch Case/3 -> If Action Subsystem2/Action
  Switch Case/2 -> If Action Subsystem7/Action
  Switch Case/1 -> If Action Subsystem8/Action
  In1/1 -> Switch Case/1

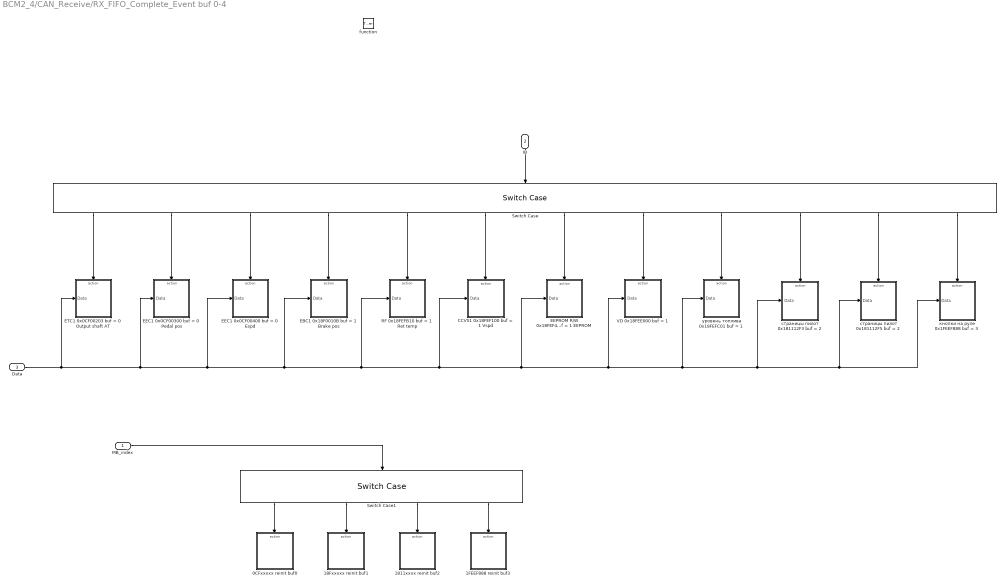
== system BCM2_4/CAN_Receive/RX_FIFO_Complete_Event buf 0-4 ==
  MB_index : Inport
  ID : Inport  Port=2
  Data : Inport  Port=3
  function : TriggerPort  TriggerType=function-call  VariantControl=Variant
  0CFxxxxx reinit buf0 : Subsystem  TreatAsAtomicUnit=on
  1811xxxx reinit buf2 : Subsystem  TreatAsAtomicUnit=on
  18Fxxxxx reinit buf1 : Subsystem  TreatAsAtomicUnit=on
  1FEEF888 reinit buf3 : Subsystem  TreatAsAtomicUnit=on
  CCVS1 0x18FEF100 buf = 1 Vspd : Subsystem  TreatAsAtomicUnit=on
  EBC1 0x18F0010B buf = 1 Brake pos : Subsystem  TreatAsAtomicUnit=on
  EEC1 0x0CF00300 buf = 0 Pedal pos : Subsystem  TreatAsAtomicUnit=on
  EEC1 0x0CF00400 buf = 0 Espd : Subsystem  TreatAsAtomicUnit=on
  EEPROM R/W 0x18FEF460 buf = 1 EEPROM : Subsystem  TreatAsAtomicUnit=on
  ETC1 0x0CF00203 buf = 0 Output shaft AT : Subsystem  TreatAsAtomicUnit=on
  RF 0x18FEFB10 buf = 1 Ret temp : Subsystem  TreatAsAtomicUnit=on
  Switch Case : SwitchCase  CaseConditions={hex2dec('0CF00203'),hex2dec('0CF00300'),hex2dec('0CF00400'),hex2dec('18F0010B'),hex2dec('18FEFB10'),hex2dec('18FEF100'),hex2dec('18FEF460'),hex2dec('18FEE000'),hex2dec('18FEFC01'),hex2dec('181112F3'),hex2dec('181112F5'),hex2dec('1FEEF888') }  ShowDefaultCase=off
  Switch Case1 : SwitchCase  CaseConditions={0 1 2 3}  ShowDefaultCase=off
  VD 0x18FEE000 buf = 1 : Subsystem  TreatAsAtomicUnit=on
  кнопки на руле 0х1FEEF888 buf = 3 : Subsystem  TreatAsAtomicUnit=on
  страницы пилот 0х181112F3 buf = 2 : Subsystem  TreatAsAtomicUnit=on
  страницы пилот 0х181112F5 buf = 2 : Subsystem  TreatAsAtomicUnit=on
  уровень топлива 0х18FEFC01 buf = 1 : Subsystem  TreatAsAtomicUnit=on
  wires:
  ID/1 -> Switch Case/1
  MB_index/1 -> Switch Case1/1
  Switch Case1/1 -> 0CFxxxxx reinit buf0/Action
  Switch Case1/2 -> 18Fxxxxx reinit buf1/Action
  Switch Case/1 -> ETC1 0x0CF00203 buf = 0 Output shaft AT/Action
  Switch Case/2 -> EEC1 0x0CF00300 buf = 0 Pedal pos/Action
  Switch Case/3 -> EEC1 0x0CF00400 buf = 0 Espd/Action
  Switch Case/4 -> EBC1 0x18F0010B buf = 1 Brake pos/Action
  Switch Case/5 -> RF 0x18FEFB10 buf = 1 Ret temp/Action
  Switch Case/6 -> CCVS1 0x18FEF100 buf = 1 Vspd/Action
  Switch Case/7 -> EEPROM R/W 0x18FEF460 buf = 1 EEPROM/Action
  Data/1 -> VD 0x18FEE000 buf = 1/1(Data), уровень топлива 0х18FEFC01 buf = 1/1(Data), кнопки на руле 0х1FEEF888 buf = 3/1(Data), страницы пилот 0х181112F5 buf = 2/1(Data), страницы пилот 0х181112F3 buf = 2/1(Data), EEPROM R/W 0x18FEF460 buf = 1 EEPROM/1(Data), CCVS1 0x18FEF100 buf = 1 Vspd/1(Data), RF 0x18FEFB10 buf = 1 Ret temp/1(Data), EBC1 0x18F0010B buf = 1 Brake pos/1(Data), EEC1 0x0CF00400 buf = 0 Espd/1(Data), EEC1 0x0CF00300 buf = 0 Pedal pos/1(Data), ETC1 0x0CF00203 buf = 0 Output shaft AT/1(Data)
  Switch Case/8 -> VD 0x18FEE000 buf = 1/Action
  Switch Case/9 -> уровень топлива 0х18FEFC01 buf = 1/Action
  Switch Case1/3 -> 1811xxxx reinit buf2/Action
  Switch Case/10 -> страницы пилот 0х181112F3 buf = 2/Action
  Switch Case/11 -> страницы пилот 0х181112F5 buf = 2/Action
  Switch Case/12 -> кнопки на руле 0х1FEEF888 buf = 3/Action
  Switch Case1/4 -> 1FEEF888 reinit buf3/Action

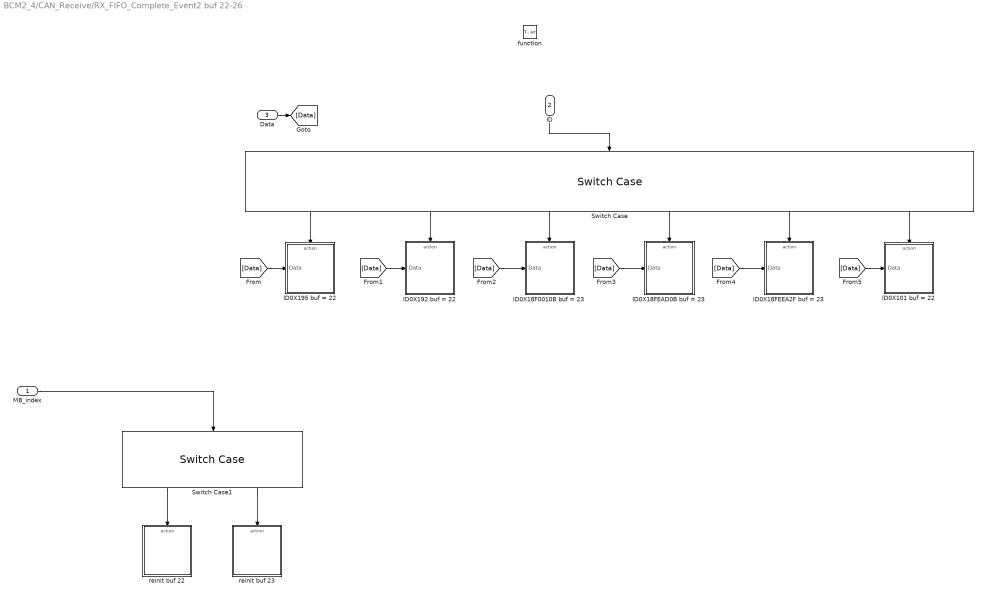
== system BCM2_4/CAN_Receive/RX_FIFO_Complete_Event2 buf 22-26 ==
  MB_index : Inport
  ID : Inport  Port=2
  Data : Inport  Port=3
  function : TriggerPort  TriggerType=function-call  VariantControl=Variant
  ID0X101 buf = 22 : Subsystem  TreatAsAtomicUnit=on
  ID0X18F0010B buf = 23 : Subsystem  TreatAsAtomicUnit=on
  ID0X18FEAD0B buf = 23 : Subsystem  TreatAsAtomicUnit=on
  ID0X18FEEA2F buf = 23 : Subsystem  TreatAsAtomicUnit=on
  ID0X192 buf = 22 : Subsystem  TreatAsAtomicUnit=on
  ID0X195 buf = 22 : Subsystem  TreatAsAtomicUnit=on
  Switch Case : SwitchCase  CaseConditions={hex2dec('195') hex2dec('192') hex2dec('18F0010B') hex2dec('18FEAD0B') hex2dec('18FEEA2F') hex2dec('101')}  ShowDefaultCase=off
  Switch Case1 : SwitchCase  CaseConditions={22 23}  ShowDefaultCase=off
  reinit buf 22 : Subsystem  TreatAsAtomicUnit=on
  reinit buf 23 : Subsystem  TreatAsAtomicUnit=on
  wires:
  [Data] -> ID0X192 buf = 22/1(Data)
  [Data] -> ID0X195 buf = 22/1(Data)
  Data/1 -> [Data]
  ID/1 -> Switch Case/1
  Switch Case/1 -> ID0X195 buf = 22/Action
  Switch Case/2 -> ID0X192 buf = 22/Action
  MB_index/1 -> Switch Case1/1
  Switch Case1/1 -> reinit buf 22/Action
  Switch Case1/2 -> reinit buf 23/Action
  Switch Case/3 -> ID0X18F0010B buf = 23/Action
  [Data] -> ID0X18F0010B buf = 23/1(Data)
  [Data] -> ID0X18FEAD0B buf = 23/1(Data)
  [Data] -> ID0X18FEEA2F buf = 23/1(Data)
  Switch Case/4 -> ID0X18FEAD0B buf = 23/Action
  Switch Case/5 -> ID0X18FEEA2F buf = 23/Action
  [Data] -> ID0X101 buf = 22/1(Data)
  Switch Case/6 -> ID0X101 buf = 22/Action

== system BCM2_4/CAN_Receive/RX_FIFO_Complete_Event3 buf 44-48 ==
  MB_index : Inport
  ID : Inport  Port=2
  Data : Inport  Port=3
  function : TriggerPort  TriggerType=function-call  VariantControl=Variant
  ID0X192 buf = 15 : Subsystem  TreatAsAtomicUnit=on
  ID0X195 buf = 15 : Subsystem  TreatAsAtomicUnit=on
  Switch Case : SwitchCase  CaseConditions={hex2dec('195') hex2dec('192')}  ShowDefaultCase=off
  Switch Case1 : SwitchCase  CaseConditions={15}  ShowDefaultCase=off
  reinit buf 15 : Subsystem  TreatAsAtomicUnit=on
  wires:
  Switch Case1/1 -> reinit buf 15/Action
  MB_index/1 -> Switch Case1/1
  Switch Case/2 -> ID0X192 buf = 15/Action
  Switch Case/1 -> ID0X195 buf = 15/Action
  ID/1 -> Switch Case/1
  Data/1 -> [Data]
  [Data] -> ID0X195 buf = 15/1(Data)
  [Data] -> ID0X192 buf = 15/1(Data)

== system BCM2_4/Drivers/Diagnostic1 ==
  Trigger : TriggerPort  TriggerType=function-call  VariantControl=Variant  PortDimensions=1
  Data Store Read3 : DataStoreRead  DataStoreName=spi_rcv_tle82453  IndexOptions=Index vector (dialog)  Indices=1  OutputSizes=1
  Selector : Selector  InputPortWidth=4  IndexOptions=Index vector (dialog)  Indices=[1:1]  OutputSizes=1
  Selector1 : Selector  InputPortWidth=4  IndexOptions=Index vector (dialog)  Indices=[2:4]  OutputSizes=1
  Switch Case : SwitchCase  CaseConditions={64,65,66,2}  ShowDefaultCase=off
  Switch Case Action Subsystem : Subsystem  TreatAsAtomicUnit=on
  Switch Case Action Subsystem1 : Subsystem  TreatAsAtomicUnit=on
  Switch Case Action Subsystem2 : Subsystem  TreatAsAtomicUnit=on
  Switch Case Action Subsystem3 : Subsystem  TreatAsAtomicUnit=on
  wires:
  Selector1/1 -> Switch Case Action Subsystem3/1(In1), Switch Case Action Subsystem2/1(In1), Switch Case Action Subsystem1/1(In1), Switch Case Action Subsystem/1(In1)
  Selector/1 -> Switch Case/1
  Switch Case/3 -> [FB2]
  Switch Case/2 -> [FB1]
  Switch Case/4 -> Switch Case Action Subsystem/Action
  [FB2] -> Switch Case Action Subsystem3/Action
  [FB0] -> Switch Case Action Subsystem1/Action
  Switch Case/1 -> [FB0]
  [FB1] -> Switch Case Action Subsystem2/Action
  Data Store Read3/1 -> Selector1/1, Selector/1

== system BCM2_4/Drivers/Subsystem ==
  send_spi() : Inport
  function : TriggerPort  TriggerType=function-call  VariantControl=Variant
  Data Store Write : DataStoreWrite  DataStoreName=recv_spi2  IndexOptions=Index vector (dialog)  Indices=1  OutputSizes=1
  SPI_Master_Transfer1 : mbd_mpc574x_ec_toolbox/Communication Blocks/SPI Blocks/SPI_Master_Transfer  Priority=8  InstanceNumber=2  xfermode=Non blocking  timeout=50  spi_upd=on  WhichPCS=3
      settings: SourceProductName=NXP Model-Based Design Toolbox for MPC57xx MCUs
  wires:
  SPI_Master_Transfer1/1 -> Data Store Write/1
  send_spi()/1 -> SPI_Master_Transfer1/1

== system BCM2_4/Drivers/Subsystem2 ==
  send_spi() : Inport
  function : TriggerPort  TriggerType=function-call  VariantControl=Variant
  Data Store Write : DataStoreWrite  DataStoreName=spi_rcv_tle82453  IndexOptions=Index vector (dialog)  Indices=1  OutputSizes=1
  SPI_Master_Transfer1 : mbd_mpc574x_ec_toolbox/Communication Blocks/SPI Blocks/SPI_Master_Transfer  Priority=8  InstanceNumber=1  xfermode=Non blocking  timeout=50  spi_upd=on  WhichPCS=0
      settings: SourceProductName=NXP Model-Based Design Toolbox for MPC57xx MCUs
  wires:
  send_spi()/1 -> SPI_Master_Transfer1/1
  SPI_Master_Transfer1/1 -> Data Store Write/1

== system BCM2_4/Drivers/Subsystem3 ==
  send_spi() : Inport
  function : TriggerPort  TriggerType=function-call  VariantControl=Variant
  SPI_Master_Transfer1 : mbd_mpc574x_ec_toolbox/Communication Blocks/SPI Blocks/SPI_Master_Transfer  Priority=8  InstanceNumber=1  xfermode=Non blocking  timeout=50  spi_upd=on  WhichPCS=1
      settings: SourceProductName=NXP Model-Based Design Toolbox for MPC57xx MCUs
  Terminator : Terminator
  wires:
  SPI_Master_Transfer1/1 -> Terminator/1
  send_spi()/1 -> SPI_Master_Transfer1/1

== system BCM2_4/Drivers/input status ==
  Trigger : TriggerPort  TriggerType=function-call  VariantControl=Variant  PortDimensions=1
  Data Store Read : DataStoreRead  DataStoreName=recv_spi2  DataStoreElements=recv_spi2(1)  IndexOptions=Index vector (dialog)  Indices=1  OutputSizes=1
  Data Store Read1 : DataStoreRead  DataStoreName=recv_spi2  DataStoreElements=recv_spi2(1)  IndexOptions=Index vector (dialog)  Indices=1  OutputSizes=1
  Switch Case : SwitchCase  CaseConditions="{hex2dec(\"0x3E\")}"
  Switch Case Action Subsystem : Subsystem  TreatAsAtomicUnit=on
  Switch Case Action Subsystem1 : Subsystem  TreatAsAtomicUnit=on
  Switch Case Action Subsystem2 : Subsystem  TreatAsAtomicUnit=on
  Switch Case Action Subsystem3 : Subsystem  TreatAsAtomicUnit=on
  Switch Case1 : SwitchCase  CaseConditions="{hex2dec(\"0x3E\")}"
  wires:
  Data Store Read/1 -> Switch Case/1
  Switch Case/1 -> Switch Case Action Subsystem/Action
  Switch Case/2 -> Switch Case Action Subsystem1/Action
  Switch Case1/2 -> Switch Case Action Subsystem3/Action
  Switch Case1/1 -> Switch Case Action Subsystem2/Action
  Data Store Read1/1 -> Switch Case1/1

== system BCM2_4/Drivers/mem copy read1 ==
  function : TriggerPort  TriggerType=function-call  VariantControl=Variant
  Byte Unpack : etargetslib/Byte Unpack  dimensions={[1]}  datatypes={'uint16'}  byteAlign=1
  Data Store Read : DataStoreRead  DataStoreName=ee_recv  IndexOptions=Index vector (dialog)  Indices=1  OutputSizes=1
  Data Store Write : DataStoreWrite  DataStoreName=ee_read  IndexOptions=Index vector (dialog)  Indices=1  OutputSizes=1
  Selector : Selector  InputPortWidth=5  IndexOptions=Index vector (dialog)  Indices=[4 5]  OutputSizes=1
  wires:
  Selector/1 -> Byte Unpack/1
  Data Store Read/1 -> Selector/1
  Byte Unpack/1 -> Data Store Write/1

== system BCM2_4/Drivers/send data spi1 ==
  out_data : Inport
  function : TriggerPort  TriggerType=function-call  VariantControl=Variant
  Data Store Write2 : DataStoreWrite  DataStoreName=ee_recv  IndexOptions=Index vector (dialog)  Indices=1  OutputSizes=1
  SPI_Master_Transfer : mbd_mpc574x_ec_toolbox/Communication Blocks/SPI Blocks/SPI_Master_Transfer  InstanceNumber=3  xfermode=Non blocking  timeout=50  spi_upd=on  WhichPCS=0
  wires:
  SPI_Master_Transfer/1 -> Data Store Write2/1
  out_data/1 -> SPI_Master_Transfer/1

== system BCM2_4/Drivers/write cmd eeprom1 ==
  function : TriggerPort  TriggerType=function-call  VariantControl=Variant
  Constant : Constant  Value=6  OutDataTypeStr=uint8
  SPI_Master_Transfer : mbd_mpc574x_ec_toolbox/Communication Blocks/SPI Blocks/SPI_Master_Transfer  InstanceNumber=3  xfermode=Non blocking  timeout=50  spi_upd=on  WhichPCS=0
  Terminator : Terminator
  wires:
  SPI_Master_Transfer/1 -> Terminator/1
  Constant/1 -> SPI_Master_Transfer/1

== system BCM2_4/Init System/Начальная иницилизация ==
  Constant13 : Constant  Value=[0.32 0.36 0.41 0.44 0.5 0.6]  OutDataTypeStr=double  SampleTime=-1
  Data Store Write : DataStoreWrite  DataStoreName=ret  DataStoreElements=ret.stepM(:)  IndexOptions=Index vector (dialog)  Indices=1  OutputSizes=1
  Event Listener : EventListener  DisableCoverage=on  EventName=reset
  Init filters CAN : Subsystem
  wires:
  Constant13/1 -> Data Store Write/1
